simulink model "CartesianCB"  (Simulink 7.1)
settings: Solver=ode45  SolverMode=SingleTasking  StartTime=0.0  StopTime=10.0  RelTol=1e-3  AbsTol=1e-6
settings Model: Creator=The MathWorks Inc.  LastModifiedBy=suarezjl  ExtModeTrigMode=oneshot  ExtModeArmWhenConnect=off  ExtModeAutoUpdateStatusClock=off
settings DataIOCC: LimitDataPoints=off  SignalLoggingName=logsOut
settings OptimizationCC: BooleanDataType=off  InlineInvariantSignals=on
settings DebuggingCC: SaveWithParameterizedLinksMsg=none  CheckExecutionContextPreStartOutputMsg=on  CheckExecutionContextRuntimeOutputMsg=on  SignalResolutionControl=TryResolveAllWithWarning  SolverPrmCheckMsg=none  MultiTaskDSMMsg=warning  MultiTaskCondExecSysMsg=none  IntegerOverflowMsg=none  StrictBusMsg=None
settings HardwareCC: TargetUnknown=on
settings ModelReferenceCC: UpdateModelReferenceTargets=IfOutOfDate
settings RTWCC: IncludeERTFirstTime=on
settings GRTTargetCC: TargetFcnLib=ansi_tfl_tmw.mat

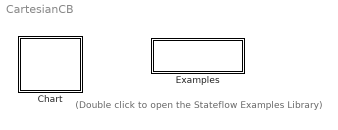
== system CartesianCB ==
  note: (Double click to open the
      | Stateflow Examples Library)
  Chart : Stateflow chart
  Examples : Subsystem
      settings: OpenFcn=sf('Private','sf_examples')
      mask Display: disp('Examples')

== system CartesianCB/Examples ==

== stateflow chart Chart ==
  state Initialize
    Aquateen\ControlBasisModuleC\CartesianCB\CartesianCB.Initialize()
    Aquateen\ControlBasisModuleC\HP3JCAgent\HP3JC.connect_Initialize()
    Aquateen\ControlBasisModuleC\HP3JCAgent\HP3JC.servo_ServoOn()
    Aquateen\ControlBasisModuleC\HP3JCAgent\HP3JC.job_SelectJob()
    Aquateen\ControlBasisModuleC\HP3JCAgent\HP3JC.job_StartJob()
  state ReadPosition
    Aquateen\ControlBasisModuleC\HP3JCAgent\HP3JC.read_CurrentPosition()
    Aquateen\ControlBasisModuleC\CartesianCB\CartesianCB.ComputeControlBasis()
    Aquateen\ControlBasisModuleC\HP3JCAgent\move__LinearMotion()
  state Stop
    Aquateen\ControlBasisModuleC\HP3JCAgent\HP3JC.error_ClearError()
    Aquateen\ControlBasisModuleC\HP3JCAgent\HP3JC.error_ClearAlarm()
    Aquateen\ControlBasisModuleC\HP3JCAgent\HP3JC.job_SelectJob()
    Aquateen\ControlBasisModuleC\HP3JCAgent\HP3JC.job_StartJob()
    Aquateen\ControlBasisModuleC\HP3JCAgent\HP3JC.job_StartJob()
    Aquateen\ControlBasisModuleC\IKinControlBasis\StateMachine.Wait(2000)
    Aquateen\ControlBasisModuleC\HP3JCAgent\HP3JC.connect_Disconnect()
  (default) -> Initialize : Start
  Initialize -> ReadPosition : Always
  ReadPosition -> ReadPosition [order 1] : Default
  ReadPosition -> Stop [order 2] : Signal="Stop"
